simulink model "system_SOLENOID_working_temp"  (R2018a)
settings: Solver=ode15s  StartTime=0.0  StopTime=150  MaxStep=1e-3  RelTol=1e-3
InitFcn:
  | params_SMA
undefined symbols (not defined in the file or in its folder): fluid, solenoid, valve
libraries: simulink x1
settings Model: Creator=Felix Welsch  LastModifiedBy=tim
settings OptimizationCC: LifeSpan=inf
settings DebuggingCC: SFExecutionAtInitializationDiag=none
settings CodeAppCC: StateflowObjectComments=on

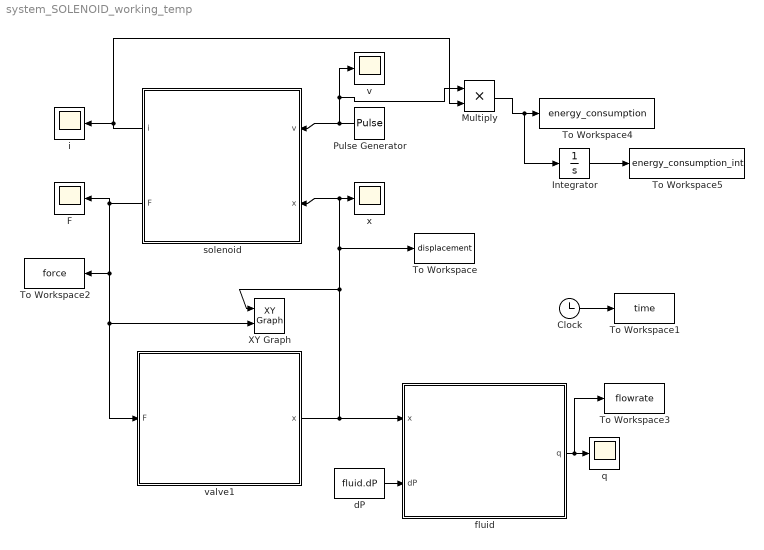
== system system_SOLENOID_working_temp ==
  Clock : Clock
  F : Scope
  Integrator : Integrator
  Multiply : Product
  Pulse Generator : DiscretePulseGenerator  PulseType=Time based  Amplitude=12  Period=10  PulseWidth=50  PhaseDelay=2.5
  To Workspace : ToWorkspace  VariableName=displacement  SampleTime=-1
  To Workspace1 : ToWorkspace  VariableName=time  SampleTime=-1
  To Workspace2 : ToWorkspace  VariableName=force  SampleTime=-1
  To Workspace3 : ToWorkspace  VariableName=flowrate  SampleTime=-1
  To Workspace4 : ToWorkspace  VariableName=energy_consumption  SampleTime=-1
  To Workspace5 : ToWorkspace  VariableName=energy_consumption_int  SampleTime=-1
  XY Graph : simulink/Sinks/XY Graph  xmin=0  xmax=7e-3  ymin=0  ymax=10  st=-1
  dP : Constant  Value=fluid.dP
  fluid : Subsystem
  i : Scope
  q : Scope
  solenoid : Subsystem
  "v " : Scope
  valve1 : Subsystem
  x : Scope
  wires:
  fluid/1(q) -> To Workspace3/1, q/1
  dP/1 -> fluid/2(dP)
  solenoid/1(i) -> Multiply/2, i/1
  Pulse Generator/1 -> solenoid/1(v), Multiply/1, "v "/1
  solenoid/2(F) -> F/1, To Workspace2/1, valve1/1(F), XY Graph/2
  Clock/1 -> To Workspace1/1
  valve1/1(x) -> fluid/1(x), To Workspace/1, x/1, solenoid/2(x), XY Graph/1
  Multiply/1 -> Integrator/1, To Workspace4/1
  Integrator/1 -> To Workspace5/1

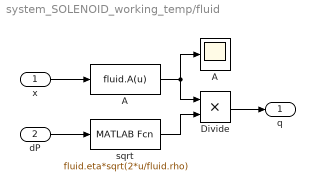
== system system_SOLENOID_working_temp/fluid ==
  x : Inport
  dP : Inport  Port=2
  A : MATLABFcn  MATLABFcn=fluid.A(u)
  "A " : Scope
  Divide : Product  Inputs=**
  sqrt : MATLABFcn  MATLABFcn=fluid.eta*sqrt(2*u/fluid.rho)
  q : Outport
  wires:
  x/1 -> A/1
  dP/1 -> sqrt/1
  A/1 -> "A "/1, Divide/1
  sqrt/1 -> Divide/2
  Divide/1 -> q/1

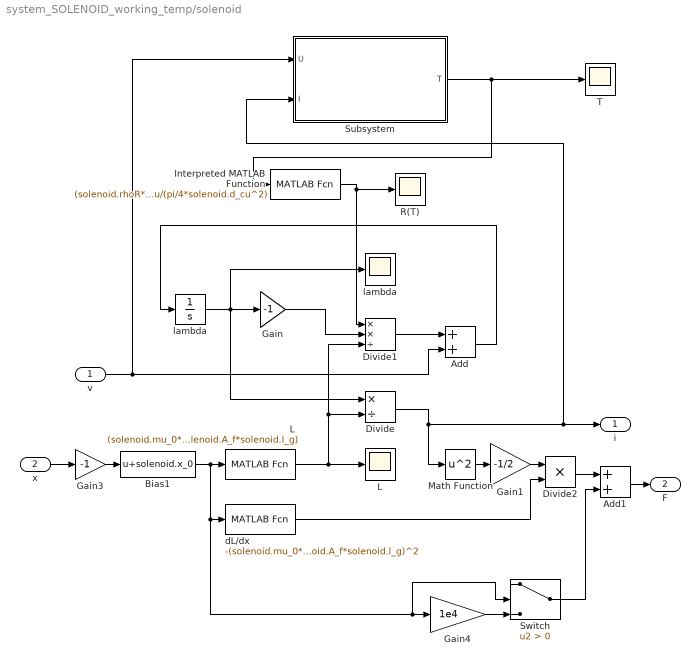
== system system_SOLENOID_working_temp/solenoid ==
  v : Inport
  x : Inport  Port=2
  Add : Sum
  Add1 : Sum
  Bias1 : Bias  Bias=solenoid.x_0
  Divide : Product  Inputs=*/
  Divide1 : Product  Inputs=**/
  Divide2 : Product  Inputs=**
  Gain : Gain  Gain=-1
  Gain1 : Gain  Gain=-1/2
  Gain3 : Gain  Gain=-1
  Gain4 : Gain  Gain=1e4
  Interpreted MATLAB Function : MATLABFcn  MATLABFcn=(solenoid.rhoR*(1+solenoid.alphaR*(u-solenoid.T0R)))*solenoid.l_cu/(pi/4*solenoid.d_cu^2)
  L : MATLABFcn  MATLABFcn=(solenoid.mu_0*solenoid.A_f*solenoid.A_g*solenoid.N^2) / (solenoid.A_g*u+solenoid.A_f*solenoid.l_g)
  "L " : Scope
  Math Function : Math  Operator=square  SaturateOnIntegerOverflow=on
  R(T) : Scope
  Subsystem : Subsystem
  Switch : Switch  Criteria=u2 > Threshold
  T : Scope
  dL/dx : MATLABFcn  MATLABFcn=-(solenoid.mu_0*solenoid.A_f*solenoid.A_g*solenoid.N^2*solenoid.A_g) / (solenoid.A_g*u+solenoid.A_f*solenoid.l_g)^2
  lambda : Integrator
  "lambda " : Scope
  i : Outport
  F : Outport  Port=2
  wires:
  Add/1 -> lambda/1
  Divide1/1 -> Add/1
  Gain1/1 -> Divide2/1
  lambda/1 -> "lambda "/1, Gain/1, Divide/1
  Divide/1 -> Math Function/1, Subsystem/2(I), i/1
  x/1 -> Gain3/1
  L/1 -> "L "/1, Divide1/3, Divide/2
  Math Function/1 -> Gain1/1
  dL/dx/1 -> Divide2/2
  Gain/1 -> Divide1/2
  v/1 -> Subsystem/1(U), Add/2
  Interpreted MATLAB Function/1 -> R(T)/1, Divide1/1
  Gain3/1 -> Bias1/1
  Bias1/1 -> Gain4/1, Switch/2, dL/dx/1, L/1
  Gain4/1 -> Switch/3
  Divide2/1 -> Add1/1
  Switch/1 -> Add1/2
  Add1/1 -> F/1
  Subsystem/1(T) -> Interpreted MATLAB Function/1, T/1

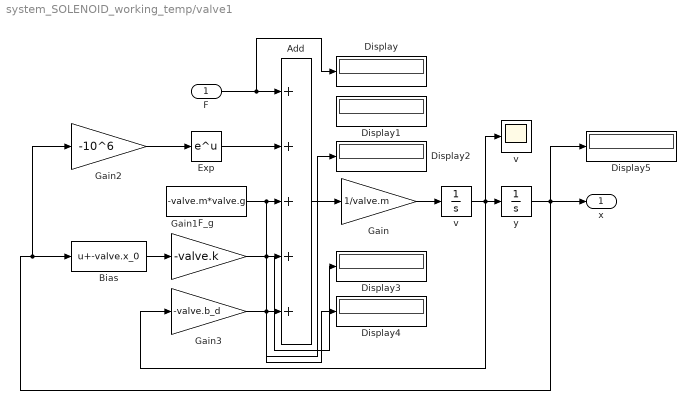
== system system_SOLENOID_working_temp/valve1 ==
  F : Inport
  Add : Sum  Inputs=+++++
  Bias : Bias  Bias=-valve.x_0
  Display{,1..5} (6 alike) : Display
  Exp : Math  SaturateOnIntegerOverflow=on
  F_g : Constant  Value=-valve.m*valve.g
  Gain : Gain  Gain=1/valve.m
  Gain1 : Gain  Gain=-valve.k
  Gain2 : Gain  Gain=-10^6
  Gain3 : Gain  Gain=-valve.b_d
  v : Integrator  InitialCondition=valve.v_0
  "v " : Scope
  y : Integrator  InitialCondition=valve.y_0
  x : Outport
  wires:
  F_g/1 -> Display2/1, Add/3
  y/1 -> Display5/1, x/1, Gain2/1, Bias/1
  v/1 -> "v "/1, Gain3/1, y/1
  Bias/1 -> Gain1/1
  Add/1 -> Gain/1
  Gain/1 -> v/1
  F/1 -> Display/1, Add/1
  Gain1/1 -> Display3/1, Add/4
  Gain3/1 -> Display4/1, Add/5
  Exp/1 -> Add/2
  Gain2/1 -> Exp/1

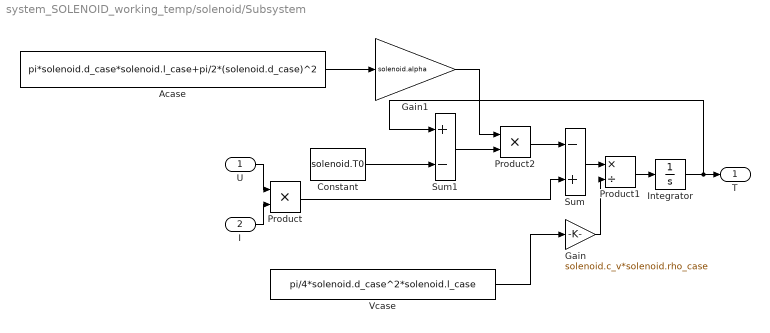
== system system_SOLENOID_working_temp/solenoid/Subsystem ==
  U : Inport
  I : Inport  Port=2
  Acase : Constant  Value=pi*solenoid.d_case*solenoid.l_case+pi/2*(solenoid.d_case)^2
  Constant : Constant  Value=solenoid.T0
  Gain : Gain  Gain=solenoid.c_v*solenoid.rho_case
  Gain1 : Gain  Gain=solenoid.alpha
  Integrator : Integrator  InitialCondition=solenoid.T0
  Product : Product
  Product1 : Product  Inputs=*/
  Product2 : Product
  Sum : Sum  Inputs=-+
  Sum1 : Sum  Inputs=+-
  "Vcase " : Constant  Value=pi/4*solenoid.d_case^2*solenoid.l_case
  T : Outport
  wires:
  Integrator/1 -> Sum1/1, T/1
  I/1 -> Product/2
  U/1 -> Product/1
  Product1/1 -> Integrator/1
  Sum/1 -> Product1/1
  Product/1 -> Sum/2
  "Vcase "/1 -> Gain/1
  Gain/1 -> Product1/2
  Product2/1 -> Sum/1
  Sum1/1 -> Product2/2
  Acase/1 -> Gain1/1
  Gain1/1 -> Product2/1
  Constant/1 -> Sum1/2
